simulink model "spacecraft_attitude_model"  (R2024b)
settings: Solver=ode4  StartTime=t0  StopTime=tf  FixedStep=0.1  RelTol=1e-3
values from neighbouring files (symbols this model uses):
  a = (((T/(2*pi))^2*mu_earth)^(1/3))    (= 7069867.85099)    [main_spacecraft_attitude_dynamics.m]
  A_body1 = surface(1)    [main_spacecraft_attitude_dynamics.m]
  A_body2 = surface(2)    [main_spacecraft_attitude_dynamics.m]
  A_body3 = surface(3)    [main_spacecraft_attitude_dynamics.m]
  A_body4 = surface(4)    [main_spacecraft_attitude_dynamics.m]
  A_body5 = surface(5)    [main_spacecraft_attitude_dynamics.m]
  A_body6 = surface(6)    [main_spacecraft_attitude_dynamics.m]
  A_panel1 = surface(7)    [main_spacecraft_attitude_dynamics.m]
  A_panel2 = surface(8)    [main_spacecraft_attitude_dynamics.m]
  A_panel3 = surface(9)    [main_spacecraft_attitude_dynamics.m]
  A_panel4 = surface(10)    [main_spacecraft_attitude_dynamics.m]
  alpha = [alpha1,alpha2,alpha3]    [main_spacecraft_attitude_dynamics.m]
  Ap = pinv(Ar)    [main_spacecraft_attitude_dynamics.m]
  Ar = Ar./norm(Ar)    [main_spacecraft_attitude_dynamics.m]
  AtmosphereModel = struct()    [AtmosphereData.m]    (also in main_spacecraft_attitude_dynamics.m)
  CD = 2.6    [main_spacecraft_attitude_dynamics.m]
  D_max = 50    [main_spacecraft_attitude_dynamics.m]
  Detumbling_time = 5000    [main_spacecraft_attitude_dynamics.m]
  e = 0.001    [main_spacecraft_attitude_dynamics.m]
  FOV = 128 * pi/180    (= 2.23402144255)    [main_spacecraft_attitude_dynamics.m]
  g1_0 = DGRF2020(1).g_nm    [main_spacecraft_attitude_dynamics.m]
  g1_1 = DGRF2020(2).g_nm    [main_spacecraft_attitude_dynamics.m]
  H = 700    [main_spacecraft_attitude_dynamics.m]
  h0 = 0    [main_spacecraft_attitude_dynamics.m]
  h1_1 = DGRF2020(2).h_nm    [main_spacecraft_attitude_dynamics.m]
  i = deg2rad(98.18)    [main_spacecraft_attitude_dynamics.m]
  Ir = 0.1    [main_spacecraft_attitude_dynamics.m]
  J = EXTRACTED_DATA.I_total    [main_spacecraft_attitude_dynamics.m]
  j_B = [0.01, 0.05, 0.01]'    [main_spacecraft_attitude_dynamics.m]
  k1 = max(max(kd_slew))    [main_spacecraft_attitude_dynamics.m]
  k2 = max(max(kp_slew))    [main_spacecraft_attitude_dynamics.m]
  Kw = max(max(kp_detumbling))    [main_spacecraft_attitude_dynamics.m]
  n = sqrt((G*M_E)/(r_earth^3))    [main_spacecraft_attitude_dynamics.m]
  N_B1 = N_B(1, :)'    [main_spacecraft_attitude_dynamics.m]
  N_B2 = N_B(2, :)'    [main_spacecraft_attitude_dynamics.m]
  N_B3 = N_B(3, :)'    [main_spacecraft_attitude_dynamics.m]
  N_B4 = N_B(4, :)'    [main_spacecraft_attitude_dynamics.m]
  N_B5 = N_B(5, :)'    [main_spacecraft_attitude_dynamics.m]
  N_B6 = N_B(6, :)'    [main_spacecraft_attitude_dynamics.m]
  N_P1 = N_B(7, :)'    [main_spacecraft_attitude_dynamics.m]
  N_P2 = N_B(8, :)'    [main_spacecraft_attitude_dynamics.m]
  N_P3 = N_B(9, :)'    [main_spacecraft_attitude_dynamics.m]
  N_P4 = N_B(10, :)'    [main_spacecraft_attitude_dynamics.m]
  n_S = (2*pi)/T_S    (= 1.99238499086e-07)    [main_spacecraft_attitude_dynamics.m]
  om = deg2rad(0)    [main_spacecraft_attitude_dynamics.m]
  P = Fe/c    (= 4.52980041279e-06)    [main_spacecraft_attitude_dynamics.m]
  pd_body1 = rho_D(1)    [main_spacecraft_attitude_dynamics.m]
  pd_body2 = rho_D(2)    [main_spacecraft_attitude_dynamics.m]
  pd_body3 = rho_D(3)    [main_spacecraft_attitude_dynamics.m]
  pd_body4 = rho_D(4)    [main_spacecraft_attitude_dynamics.m]
  pd_body5 = rho_D(5)    [main_spacecraft_attitude_dynamics.m]
  pd_body6 = rho_D(6)    [main_spacecraft_attitude_dynamics.m]
  pd_panel1 = rho_D(7)    [main_spacecraft_attitude_dynamics.m]
  pd_panel2 = rho_D(8)    [main_spacecraft_attitude_dynamics.m]
  pd_panel3 = rho_D(9)    [main_spacecraft_attitude_dynamics.m]
  pd_panel4 = rho_D(10)    [main_spacecraft_attitude_dynamics.m]
  ps_body1 = rho_S(1)    [main_spacecraft_attitude_dynamics.m]
  ps_body2 = rho_S(2)    [main_spacecraft_attitude_dynamics.m]
  ps_body3 = rho_S(3)    [main_spacecraft_attitude_dynamics.m]
  ps_body4 = rho_S(4)    [main_spacecraft_attitude_dynamics.m]
  ps_body5 = rho_S(5)    [main_spacecraft_attitude_dynamics.m]
  ps_body6 = rho_S(6)    [main_spacecraft_attitude_dynamics.m]
  ps_panel1 = rho_S(7)    [main_spacecraft_attitude_dynamics.m]
  ps_panel2 = rho_S(8)    [main_spacecraft_attitude_dynamics.m]
  ps_panel3 = rho_S(9)    [main_spacecraft_attitude_dynamics.m]
  ps_panel4 = rho_S(10)    [main_spacecraft_attitude_dynamics.m]
  q0 = [q1_0 q2_0 q3_0 q4_0]    [main_spacecraft_attitude_dynamics.m]
  r_earth = (R_earth + H)*10^3    (= 7078136.3)    [main_spacecraft_attitude_dynamics.m]
  R_earth = 6378.1363    [main_spacecraft_attitude_dynamics.m]
  r_f1 = r_F(1, :)'    [main_spacecraft_attitude_dynamics.m]
  r_f10 = r_F(10, :)'    [main_spacecraft_attitude_dynamics.m]
  r_f2 = r_F(2, :)'    [main_spacecraft_attitude_dynamics.m]
  r_f3 = r_F(3, :)'    [main_spacecraft_attitude_dynamics.m]
  r_f4 = r_F(4, :)'    [main_spacecraft_attitude_dynamics.m]
  r_f5 = r_F(5, :)'    [main_spacecraft_attitude_dynamics.m]
  r_f6 = r_F(6, :)'    [main_spacecraft_attitude_dynamics.m]
  r_f7 = r_F(7, :)'    [main_spacecraft_attitude_dynamics.m]
  r_f8 = r_F(8, :)'    [main_spacecraft_attitude_dynamics.m]
  r_f9 = r_F(9, :)'    [main_spacecraft_attitude_dynamics.m]
  r_Sun = 149597870    [main_spacecraft_attitude_dynamics.m]
  RAAN = deg2rad(RAAN)    [main_spacecraft_attitude_dynamics.m]
  sigma_b = RRW*(pi/180)*(1/3600)*(1/sqrt(Ts))    [main_spacecraft_attitude_dynamics.m]
  sigma_mag = 10^-6    (= 1e-06)    [main_spacecraft_attitude_dynamics.m]
  sigma_n = ARW*(pi/180)*(1/60)*(1/sqrt(Ts))    [main_spacecraft_attitude_dynamics.m]
  T_coil_max = 50 * 45*10^-6    (= 0.00225)    [main_spacecraft_attitude_dynamics.m]
  th0 = 0    [main_spacecraft_attitude_dynamics.m]
  v0 = [0 0 0]    [main_spacecraft_attitude_dynamics.m]
  variance_Ss = (a_sun)^2    (= 3.24)    [main_spacecraft_attitude_dynamics.m]
  w_0 = [-3, 3, 3]'    [main_spacecraft_attitude_dynamics.m]
  w_E = (2*pi)/(24*60*60)    (= 7.27220521664e-05)    [main_spacecraft_attitude_dynamics.m]
  w_LN = [0 0 0]'    [main_spacecraft_attitude_dynamics.m]
undefined symbols (not defined in the file or in its folder): A_Ss_orienation
libraries: matrix_library x38, slpidlib x2, aerolibutil x1, vrlib x1
(part 4 of 4)

== system spacecraft_attitude_model/Slew & Pointing/Subsystem/Magnetic coils/Subsystem2 ==
  T_z : Inport
  b_z : Inport  Port=2
  b_norm^2 : Inport  Port=3
  Divide2 : Product  Inputs=*/
  Product : Product
  Product1 : Product
  Saturation2 : Saturate  UpperLimit=T_coil_max  LowerLimit=-T_coil_max
  Saturation3 : Saturate  UpperLimit=D_max  LowerLimit=-D_max
  Scope2 : Scope
  Scope3 : Scope
  T_coil_z : Outport
  wires:
  Saturation3/1 -> Product1/1
  Divide2/1 -> Scope3/1, Saturation3/1
  Product/1 -> Divide2/1
  Product1/1 -> Saturation2/1
  b_norm^2/1 -> Divide2/2
  b_z/1 -> Product1/2, Product/2
  T_z/1 -> Product/1
  Saturation2/1 -> Scope2/1, T_coil_z/1

== system spacecraft_attitude_model/Envoirment/Model/Magnetic Field/b_Ned/Norm ==
  In1 : Inport
  Demux : Demux  Outputs=3
  Sqrt : Sqrt
  Square : Math  Operator=square
  Square1 : Math  Operator=square
  Square2 : Math  Operator=square
  Sum : Sum  Inputs=|+++
  Out1 : Outport
  wires:
  Demux/3 -> Square2/1
  In1/1 -> Demux/1
  Demux/1 -> Square/1
  Demux/2 -> Square1/1
  Square/1 -> Sum/1
  Square1/1 -> Sum/2
  Square2/1 -> Sum/3
  Sum/1 -> Sqrt/1
  Sqrt/1 -> Out1/1

== matlab function spacecraft_attitude_model/Attitude_determination_Sun/MATLAB Function1 ==
  data: u input; q output
function q = quest(u)

[V,D] = eig(u);
eigenvalues = D * [1 1 1 1]';
[lambda,i] = max(real(eigenvalues));
q = real(V(:,i));

end

== matlab function spacecraft_attitude_model/Pointing error/DCM err (1)/MATLAB Function ==
  data: A input; tr output
function tr = fcn(A)

tr = trace(A);
end

== matlab function spacecraft_attitude_model/Sun Sensor /Alpha Beta1/MATLAB Function ==
  data: alpha input; alphamin output; betamin output; A output; beta input; Amat input; i output
function [alphamin,betamin,A,i] = minimum(alpha, beta, Amat)

[~,i] = min(abs(alpha)+abs(beta));
alphamin = alpha(i);
betamin = beta(i);

if i==1
    A=Amat(:,:,1);
elseif i==2
    A=Amat(:,:,2);
elseif i==3
    A=Amat(:,:,3);
elseif i==4
    A=Amat(:,:,4);
elseif i==5
    A=Amat(:,:,5);
else
    A=Amat(:,:,6);
end


end
